simulink model "addFMTestHarness"  (R2024a)
settings: configuration reference "standardSILConfiguraitonParams" (kept outside this file)
settings Model: Creator=jerem  LastModifiedBy=jerem
settings ConfigSetRef: SourceName=standardSILConfiguraitonParams  SourceLocation=Base Workspace

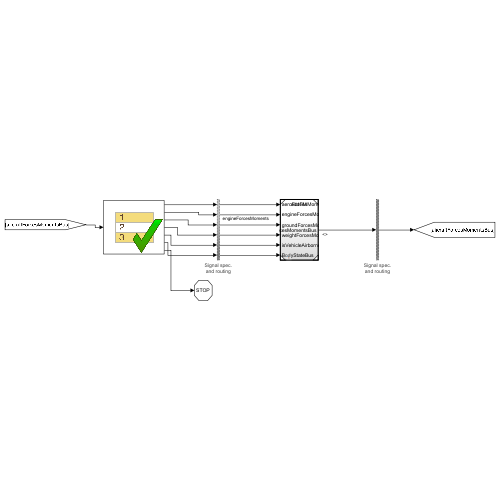
[thumbnail: Simulink's stored preview of the top-level diagram]
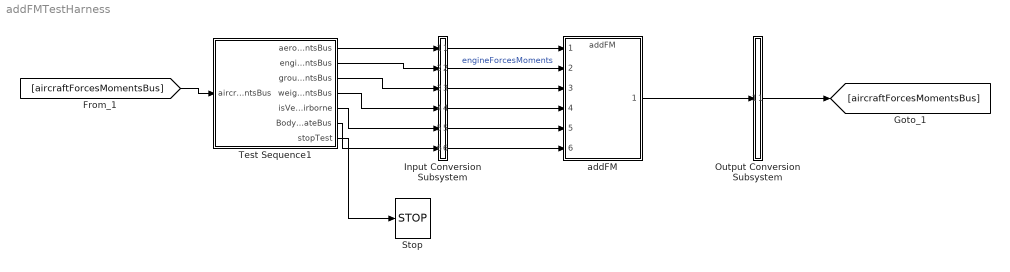
== system addFMTestHarness ==
  Input Conversion Subsystem : Subsystem  Tag=__SLT_ICS__  Description=|
      | Signal spec.
      | and routing
      settings: AttributesFormatString=%<Description>
  Output Conversion Subsystem : Subsystem  Tag=__SLT_OCS__  Description=|
      | Signal spec.
      | and routing
      mask init:
      | ICDictionary = get_param(bdroot, 'DataDictionary');
      | if isempty(ICDictionary)
      |    ICScope = Simulink.data.BaseWorkspace;
      | else
      |    ICScope = Simulink.data.DataDictionary(ICDictionary);
      | end
      | 
      | IC1 = Simulink.Bus.createMATLABStruct('AircraftForcesMomentsBus', [], [1 1], ICScope);
      settings: AttributesFormatString=%<Description>
  Stop : Stop
  Test Sequence1 : Test Sequence  TreatAsAtomicUnit=on
  addFM : ModelReference  ModelNameDialog=addFM  SimulationMode=Normal  ModelReferenceVersion=1.68
  wires:
  Test Sequence1/1(aeroForcesMomentsBus) -> Input Conversion Subsystem/1(Inport_1)
  Test Sequence1/2(engineForcesMomentsBus) -> Input Conversion Subsystem/2(Inport_2)
  Test Sequence1/3(groundForcesMomentsBus) -> Input Conversion Subsystem/3(Inport_3)
  Test Sequence1/4(weightForcesMomentsBus) -> Input Conversion Subsystem/4(Inport_4)
  [aircraftForcesMomentsBus] -> Test Sequence1/1(aircraftForcesMomentsBus)
  Output Conversion Subsystem/1(Outport_1) -> [aircraftForcesMomentsBus]
  Test Sequence1/7(stopTest) -> Stop/1
  Test Sequence1/5(isVehicleAirborne) -> Input Conversion Subsystem/5(Inport_5)
  Test Sequence1/6(BodyStateBus) -> Input Conversion Subsystem/6(Inport_6)
  addFM/1 -> Output Conversion Subsystem/1(Inport_1)
  Input Conversion Subsystem/1(Outport_1) -> addFM/1
  Input Conversion Subsystem/2(Outport_2) -> addFM/2  "engineForcesMoments"
  Input Conversion Subsystem/3(Outport_3) -> addFM/3
  Input Conversion Subsystem/4(Outport_4) -> addFM/4
  Input Conversion Subsystem/5(Outport_5) -> addFM/5
  Input Conversion Subsystem/6(Outport_6) -> addFM/6

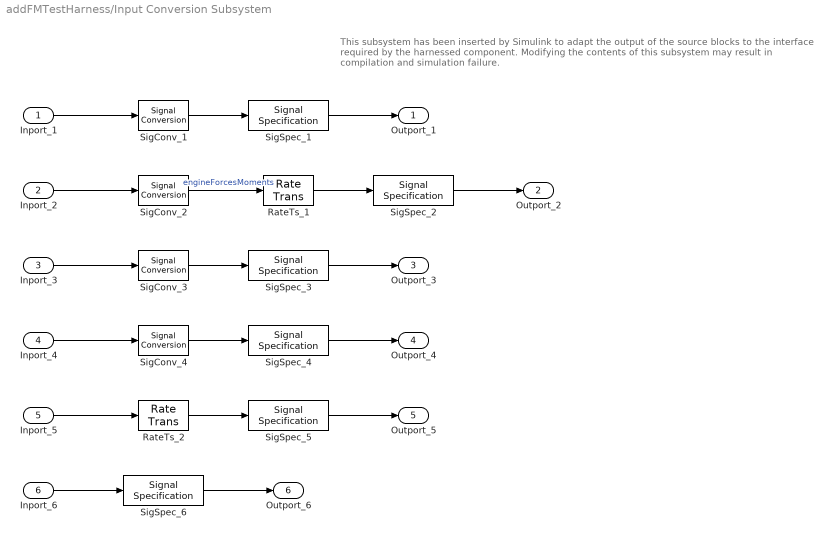
== system addFMTestHarness/Input Conversion Subsystem ==
  note: This subsystem has been inserted by Simulink to adapt the output of the source blocks to the interface required by the harnessed component.
      |  Modifying the contents of this subsystem may result in compilation and simulation failure.
  Inport_1 : Inport
  Inport_2 : Inport  Port=2
  Inport_3 : Inport  Port=3
  Inport_4 : Inport  Port=4
  Inport_5 : Inport  Port=5
  Inport_6 : Inport  Port=6
  RateTs_1 : RateTransition  OutPortSampleTime=0.004
  RateTs_2 : RateTransition  OutPortSampleTime=0.004
  SigConv_{1..4} (4 alike) : SignalConversion  ConversionOutput=Virtual bus  OverrideOpt=off
  SigSpec_1 : SignalSpecification  OutDataTypeStr=Bus: ComponentForcesMomentsBus  SampleTime=[-1, 0]
  SigSpec_2 : SignalSpecification  OutDataTypeStr=Bus: ComponentForcesMomentsBus  SampleTime=0.004
  SigSpec_3 : SignalSpecification  OutDataTypeStr=Bus: ComponentForcesMomentsBus  SampleTime=[-1, 0]
  SigSpec_4 : SignalSpecification  OutDataTypeStr=Bus: ComponentForcesMomentsBus  SampleTime=[-1, 0]
  SigSpec_5 : SignalSpecification  OutDataTypeStr=boolean  Dimensions=[1]  SampleTime=0.004
  SigSpec_6 : SignalSpecification  OutDataTypeStr=Bus: BodyStateBus  Dimensions=[1]  SampleTime=[-1, 0]  BusOutputAsStruct=on
  Outport_1 : Outport
  Outport_2 : Outport  Port=2
  Outport_3 : Outport  Port=3
  Outport_4 : Outport  Port=4
  Outport_5 : Outport  Port=5
  Outport_6 : Outport  Port=6
  wires:
  SigSpec_1/1 -> Outport_1/1
  SigConv_1/1 -> SigSpec_1/1
  Inport_1/1 -> SigConv_1/1
  SigSpec_2/1 -> Outport_2/1
  RateTs_1/1 -> SigSpec_2/1
  SigConv_2/1 -> RateTs_1/1  "engineForcesMoments"
  Inport_2/1 -> SigConv_2/1
  SigSpec_3/1 -> Outport_3/1
  SigConv_3/1 -> SigSpec_3/1
  Inport_3/1 -> SigConv_3/1
  SigSpec_4/1 -> Outport_4/1
  SigConv_4/1 -> SigSpec_4/1
  Inport_4/1 -> SigConv_4/1
  SigSpec_5/1 -> Outport_5/1
  RateTs_2/1 -> SigSpec_5/1
  Inport_5/1 -> RateTs_2/1
  SigSpec_6/1 -> Outport_6/1
  Inport_6/1 -> SigSpec_6/1

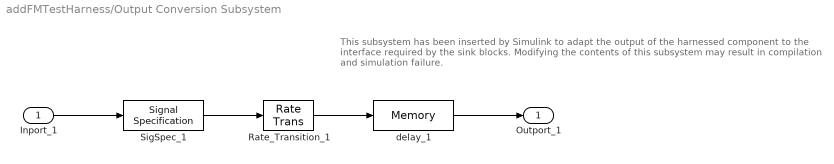
== system addFMTestHarness/Output Conversion Subsystem ==
  note: This subsystem has been inserted by Simulink to adapt the output of the harnessed component to the interface required by the sink blocks.
      |  Modifying the contents of this subsystem may result in compilation and simulation failure.
  Inport_1 : Inport
  Rate_Transition_1 : RateTransition  OutPortSampleTimeOpt=Inherit
  SigSpec_1 : SignalSpecification  OutDataTypeStr=Bus: AircraftForcesMomentsBus  Dimensions=[1]
  delay_1 : Memory  InitialCondition=IC1
  Outport_1 : Outport
  wires:
  Inport_1/1 -> SigSpec_1/1
  SigSpec_1/1 -> Rate_Transition_1/1
  Rate_Transition_1/1 -> delay_1/1
  delay_1/1 -> Outport_1/1

== stateflow chart addFMTestHarness/Test Sequence1 ==
  state Scenario_1
    state Initialize
      %% Initialize data outputs.
      stopTest = false;
      isVehicleAirborne = true;
      aeroForcesMomentsBus.forcesInBody_N = zeros(3,1);
      aeroForcesMomentsBus.momentsInBody_Nm = zeros(3,1);
      engineForcesMomentsBus.forcesInBody_N = zeros(3,1);
      engineForcesMomentsBus.momentsInBody_Nm = zeros(3,1);
      groundForcesMomentsBus.forcesInBody_N = zeros(3,1);
      groundForcesMomentsBus.momentsInBody_Nm = zeros(3,1);
      weightForcesMomentsBus.forcesInBody_N = zeros(3,1);
      weightForcesMomentsBus.momentsInBody_Nm = zeros(3,1);
      BodyStateBus.aircraftEulerAngles_rad = zeros(3,1);
      randomInputs = rand(48,1);
    state Define_Test1_Inputs
      % set to random values
      aeroForcesMomentsBus.forcesInBody_N = randomInputs(1:3);
      aeroForcesMomentsBus.momentsInBody_Nm = randomInputs(4:6);
      engineForcesMomentsBus.forcesInBody_N = randomInputs(7:9);
      engineForcesMomentsBus.momentsInBody_Nm = randomInputs(10:12);
      groundForcesMomentsBus.forcesInBody_N = randomInputs(13:15);
      groundForcesMomentsBus.momentsInBody_Nm = randomInputs(16:18);
      weightForcesMomentsBus.forcesInBody_N = randomInputs(19:21);
      weightForcesMomentsBus.momentsInBody_Nm = randomInputs(22:24);
    state Test1
      % Test 1: Check aircraftForcesMomentsBus is the sum of aeroForcesMomentsBus, engineForcesMomentsBus, and groundForcesMomentsBus
      verify(all(isClose(aircraftForcesMomentsBus.forcesInBody_N, aeroForcesMomentsBus.forcesInBody_N + engineForcesMomentsBus.forcesInBody_N + groundForcesMomentsBus.forcesInBody_N + weightForcesMomentsBus.forcesInBody_N)))
      verify(all(isClose(aircraftForcesMomentsBus.momentsInBody_Nm, engineForcesMomentsBus.momentsInBody_Nm + aeroForcesMomentsBus.momentsInBody_Nm + weightForcesMomentsBus.momentsInBody_Nm)))
    state Define_Test2_Inputs
      % set to random values
      aeroForcesMomentsBus.forcesInBody_N = randomInputs(25:27);
      aeroForcesMomentsBus.momentsInBody_Nm = randomInputs(28:30);
      engineForcesMomentsBus.forcesInBody_N = randomInputs(31:33);
      engineForcesMomentsBus.momentsInBody_Nm = randomInputs(34:36);
      groundForcesMomentsBus.forcesInBody_N = randomInputs(37:39);
      groundForcesMomentsBus.momentsInBody_Nm = randomInputs(40:42);
      weightForcesMomentsBus.forcesInBody_N = randomInputs(43:45);
      weightForcesMomentsBus.momentsInBody_Nm = randomInputs(46:48);
    state Test2
      % Test 2: Same as test 1 but with another set of random inputs
      verify(all(isClose(aircraftForcesMomentsBus.forcesInBody_N, aeroForcesMomentsBus.forcesInBody_N + engineForcesMomentsBus.forcesInBody_N + groundForcesMomentsBus.forcesInBody_N + weightForcesMomentsBus.forcesInBody_N)))
      verify(all(isClose(aircraftForcesMomentsBus.momentsInBody_Nm, aeroForcesMomentsBus.momentsInBody_Nm + engineForcesMomentsBus.momentsInBody_Nm + weightForcesMomentsBus.momentsInBody_Nm)))
    state step_1
      isVehicleAirborne = false;
    state verifyPitchIntoGround
      verify(all(isClose(aircraftForcesMomentsBus.forcesInBody_N, aeroForcesMomentsBus.forcesInBody_N + engineForcesMomentsBus.forcesInBody_N + groundForcesMomentsBus.forcesInBody_N + weightForcesMomentsBus.forcesInBody_N)))
      verify(isClose(aircraftForcesMomentsBus.momentsInBody_Nm(1), 0))
      verify(isClose(aircraftForcesMomentsBus.momentsInBody_Nm(2), engineForcesMomentsBus.momentsInBody_Nm(2) + aeroForcesMomentsBus.momentsInBody_Nm(2) + weightForcesMomentsBus.momentsInBody_Nm(2)))
      verify(isClose(aircraftForcesMomentsBus.momentsInBody_Nm(3), engineForcesMomentsBus.momentsInBody_Nm(3) + aeroForcesMomentsBus.momentsInBody_Nm(3) + weightForcesMomentsBus.momentsInBody_Nm(3)))
    state EndTest
      stopTest = true;
    (default) -> Initialize
    Initialize -> Define_Test1_Inputs : [
        | true
        | ]
    Define_Test1_Inputs -> Test1 : [
        | after(1,sec)
        | ]
    Test1 -> Define_Test2_Inputs : [
        | true
        | ]
    Define_Test2_Inputs -> Test2 : [
        | after(1,sec)
        | ]
    Test2 -> step_1 : [
        | true
        | ]
    step_1 -> verifyPitchIntoGround : [
        | after(1,sec)
        | ]
    verifyPitchIntoGround -> EndTest : [
        | true
        | ]
  (default) -> Scenario_1 : {assert(Active_Scenario_Index == 1,'The value of Scenario Parameter ''Active_Scenario_Index'' is not valid. Use the index of the scenario to specify it.')}
  data: aircraftForcesMomentsBus input Bus: AircraftForcesMomentsBus size=[1]; aeroForcesMomentsBus output Bus: ComponentForcesMomentsBus size=[1]; engineForcesMomentsBus output Bus: ComponentForcesMomentsBus size=[1]; groundForcesMomentsBus output Bus: ComponentForcesMomentsBus size=[1]; Active_Scenario_Index parameter =1; randomInputs local; weightForcesMomentsBus output Bus: ComponentForcesMomentsBus size=[1]; isVehicleAirborne output boolean; BodyStateBus output Bus: BodyStateBus; stopTest output
